simulink model "ALL_JP360_DBW_V6_5_1103"  (R2022a)
settings: Solver=FixedStepAuto  StartTime=0.0  StopTime=inf  FixedStep=0.01  RelTol=1e-3  EnableMultiTasking=on
model workspace (MAT data in the model file):
  g = 9.8
undefined symbols (not defined in the file or in its folder): canChannel, delta_v_p, IPM_Line_C0, IPM_Line_C1, IPM_Line_C2, IPM_Line_C3, M, M_p, MRR_ObjDistX, MRR_ObjDistY, MRR_ObjFusionCamID, MRR_ObjFusionSig, MRR_ObjID, MRR_ObjRelVelX, MRR_ObjRelVelY, MRR_ObjType, MRR_ObjUpdFlg, none, obj_vaild, untracktime, V, videoinput
libraries: canfdmsglib x230, canfdlib x76, slpidlib x24, simulink x18, dspstat3 x14, ctrlSharedLib x1, simulink_extras x1, imaqlib x1, realtime_pacer_lib x1, dspvision x1, visionsinks x1
(part 51 of 55)

== system ALL_JP360_DBW_V6_5_1103/ACC_Control/ACC_FUNCTION/Subsystem2/ACC_model/CC_module ==
  note: err_v＞2时根据速度段计算加速度（速度小于70mps加速度为1.5；速度大于20mps时加速度为1.3）,err_v≤2时的加速度设为0;减速度通过PID计算（速度误差0.3mps以内的减速度设为0）。
  velocity [m/s] : Inport
  Desired Velocity [m/s] : Inport  Port=2
  IC_V_kph : Inport  Port=3
  ACC_STATUSt : Inport  Port=4
  1-D Lookup Table : Lookup_n-D  NumberOfTableDimensions=1  BreakpointsForDimension1=[-2.5 -1 0 1 2 6 12 24 48 96 130]  BreakpointsForDimension2Source=Input port  Table=[-0.3 -0.1 0 0 0.8 1.5 1.7 1.8 2.0 2.0 2.2]  InternalRulePriority=Speed  RndMeth=Simplest
  1-D Lookup Table2 : Lookup_n-D  NumberOfTableDimensions=1  BreakpointsForDimension1=[-130;-96;-48;-24;-12;-6;-4;-2.5]  BreakpointsForDimension2Source=Input port  Table=[2;2;2;1;0.5;0.5;0.1;0]  InternalRulePriority=Speed  RndMeth=Simplest
  Abs2 : Abs  Commented=on  SaturateOnIntegerOverflow=off
  Add : Sum  Commented=on  Inputs=+-
  Add1 : Sum  Inputs=+-
  CalAcce : MATLAB Function  Commented=on  TreatAsAtomicUnit=on
  CalDec : slpidlib/PID Controller  Controller=PID  Form=Parallel  TimeDomain=Discrete-time  UseExternalTs=off  SampleTime=-1  IntegratorMethod=Forward Euler  FilterMethod=Forward Euler  ControllerParametersSource=external  P=1  I=1  UseKiTs=off  D=0  N=100  UseFilter=on  TunerSelectOption=Transfer Function Based (PID Tuner App)  InitialConditionSource=internal  InitialConditionForIntegrator=0  InitialConditionForFilter=0  DifferentiatorICPrevScaledInput=0  ExternalReset=either  TrackingMode=off  Kt=1  LimitOutput=off  SatLimitsSource=internal  UpperSaturationLimit=inf  LowerSaturationLimit=-inf  LinearizeAsGain=on  AntiWindupMode=none  Kb=1  POutMin=[]  POutMax=[]  IOutMin=[]  IOutMax=[]  DOutMin=[]  DOutMax=[]  NOutMin=[]  NOutMax=[]  SumOutDataTypeStr=single  SumOutMin=[]  SumOutMax=[]  SaturationOutMin=[]  SaturationOutMax=[]  PParamMin=[]  PParamMax=[]  IParamMin=[]  IParamMax=[]  DParamMin=[]  DParamMax=[]  NParamMin=[]  NParamMax=[]  KbParamMin=[]  KbParamMax=[]  KtParamMin=[]  KtParamMax=[]  KbOutMin=[]  KbOutMax=[]  KtOutMin=[]  KtOutMax=[]  IntegratorOutMin=[]  IntegratorOutMax=[]  FilterOutMin=[]  FilterOutMax=[]  SumI1OutMin=[]  SumI1OutMax=[]  SumI2OutMin=[]  SumI2OutMax=[]  SumI3OutMin=[]  SumI3OutMax=[]  SumI4OutMin=[]  SumI4OutMax=[]  SumDOutMin=[]  SumDOutMax=[]  DifferentiatorOutMin=[]  DifferentiatorOutMax=[]  FilterDiffOutCoefMin=[]  FilterDiffOutCoefMax=[]  ReciprocalOutMin=[]  ReciprocalOutMax=[]  SumDenOutMin=[]  SumDenOutMax=[]  SumNumOutMin=[]  SumNumOutMax=[]  DivideOutMin=[]  DivideOutMax=[]  UdiffTsProdOutMin=[]  UdiffTsProdOutMax=[]  NTsProdOutMin=[]  NTsProdOutMax=[]  UintegralTsProdOutMin=[]  UintegralTsProdOutMax=[]  UngainTsProdOutMin=[]  UngainTsProdOutMax=[]  IntegratorContinuousStateAttributes=''  IntegratorStateMustResolveToSignalObject=off  IntegratorRTWStateStorageClass=Auto  FilterContinuousStateAttributes=''  FilterStateMustResolveToSignalObject=off  FilterRTWStateStorageClass=Auto  ParallelPVariant=ExternalParameters  IdealPVariant=Disabled  IVariant=ExternalParameters  DVariant=ExternalParameters  IntegratorVariant=Discrete  SatVariant=Disabled  AWVariant=Passthrough  PCopyVariant=Disabled  TRVariant=Disabled  FdbkBlocksVariant=Forward  IdealPFdbkVariant=Disabled  SatFdbkVariant=Disabled  DerivativeFilterVariant=ForwardEulerFilter  NVariant=ExternalParameters  NCopyVariant=Disabled  FilterICVariant=InternalICsFilter  IntegratorICVariant=InternalICs  ExternalResetVariant=ExternalReset  TRSumVariant=Passthrough  SumFdbkVariant=Disabled  SumVariant=Sum_PID  TsampFilterVariant=InternalTs  TsampNgainVariant=Passthrough  TsampIntegralVariant=Passthrough  ExternalSaturationOutDataTypeStr=Inherit: Same as second input  aMode=0
  Constant1 : Constant  Commented=on  Value=0.01  OutDataTypeStr=single
  Constant10 : Constant  Value=100  OutDataTypeStr=int8
  Constant11 : Constant  OutDataTypeStr=single
  Constant12 : Constant  OutDataTypeStr=single
  Constant2 : Constant  Commented=on  Value=0  OutDataTypeStr=single
  Constant3 : Constant  Commented=on  Value=0  OutDataTypeStr=single
  Constant4 : Constant  Commented=on  Value=3  OutDataTypeStr=int8
  Constant{5..7,9} (4 alike) : Constant  Value=0  OutDataTypeStr=single
  Constant8 : Constant  Value=3  OutDataTypeStr=int8
  Data Type Conversion1 : DataTypeConversion  OutDataTypeStr=double  SaturateOnIntegerOverflow=off  RndMeth=Floor
  Display : Display
  From6 : From  Commented=on  GotoTag=IC_V
  Gain : Gain  Gain=3.6
  Gain1 : Gain  Gain=3.6
  Gain2 : Gain  Gain=3.6
  Gain3 : Gain  Gain=0.65
  MATLAB Function : MATLAB Function  TreatAsAtomicUnit=on
  Product : Product
  Saturation : Saturate  Commented=through  UpperLimit=1000000  LowerLimit=-10
  Saturation1 : Saturate  UpperLimit=0  LowerLimit=-2  OutDataTypeStr=single
  Saturation3 : Saturate  UpperLimit=130  LowerLimit=-2.5
  Saturation4 : Saturate  Commented=on  UpperLimit=Uplimit_acc  LowerLimit=0  OutDataTypeStr=single
  Saturation5 : Saturate  Commented=on  UpperLimit=0  LowerLimit=Uplimit_dec  OutDataTypeStr=single
  Scope : Scope  NumInputPorts=3
  Scope1 : Scope  Commented=on  NumInputPorts=3
  Sum4 : Sum  Inputs=|+-
  Switch : Switch  Threshold=-4  OutDataTypeStr=single  SaturateOnIntegerOverflow=off  InputSameDT=off
  Switch1 : Switch  Commented=on  Criteria=u2 ~= 0  SaturateOnIntegerOverflow=off  InputSameDT=off
  Switch2 : Switch  Commented=on  Criteria=u2 > Threshold  Threshold=-2.5  SaturateOnIntegerOverflow=off  InputSameDT=off
  Switch3 : Switch  Criteria=u2 ~= 0  Threshold=-0.6  SaturateOnIntegerOverflow=off  InputSameDT=off
  Switch4 : Switch  Commented=on  Criteria=u2 > Threshold  Threshold=0.3  SaturateOnIntegerOverflow=off  InputSameDT=off
  Switch5 : Switch  Threshold=-4  OutDataTypeStr=single  SaturateOnIntegerOverflow=off  InputSameDT=off
  cc_acceleration [a] : Outport
  cc_deceleration [-a] : Outport  Port=2
  wires:
  From6/1 -> CalAcce/2(IC_V)  "throttle"
  Data Type Conversion1/1 -> CalDec/1  "err_v"
  Sum4/1 -> Gain1/1, Gain/1, CalAcce/1(delta_v), Gain2/1, Saturation1/1  "err_v"
  Constant9/1 -> CalDec/4
  Constant10/1 -> CalDec/5
  velocity [m/s]/1 -> Sum4/2
  IC_V_kph/1 -> [IC_V]
  Desired Velocity [m/s]/1 -> Sum4/1
  Saturation1/1 -> Data Type Conversion1/1
  Constant2/1 -> Switch1/1
  ACC_STATUSt/1 -> [accs], Add/1
  Constant4/1 -> Add/2
  Add/1 -> Switch1/2
  Constant1/1 -> Switch1/3
  [accs] -> Add1/1
  Constant8/1 -> Add1/2
  Constant6/1 -> Switch3/1
  Product/1 -> Switch3/3  "dec"
  Add1/1 -> Switch3/2
  Switch3/1 -> MATLAB Function/3(dec_in), Display/1
  1-D Lookup Table/1 -> MATLAB Function/1(acc_in)
  ? -> Switch4/1
  Abs2/1 -> Switch4/2
  Constant3/1 -> Switch4/3
  Gain2/1 -> Switch5/2, Switch/2, 1-D Lookup Table2/1
  1-D Lookup Table2/1 -> Gain3/1
  ? -> Scope1/3
  Saturation4/1 -> Scope1/1
  Saturation5/1 -> Scope1/2
  Switch2/1 -> Saturation4/1, Saturation5/1
  Gain1/1 -> Scope/2, MATLAB Function/2(delta_v)
  MATLAB Function/1(acc_out) -> Saturation/1
  MATLAB Function/2(dec_out) -> cc_deceleration [-a]/1, Scope/3
  Gain/1 -> Saturation3/1
  Saturation3/1 -> 1-D Lookup Table/1
  Switch/1 -> CalDec/3
  Constant5/1 -> Switch/1
  Constant7/1 -> Switch/3
  Saturation/1 -> cc_acceleration [a]/1, Scope/1
  Constant12/1 -> Switch5/1
  Constant11/1 -> Switch5/3
  Switch5/1 -> Product/2
  CalDec/1 -> Product/1  "dec"
  Gain3/1 -> CalDec/2

== system ALL_JP360_DBW_V6_5_1103/ACC_Control/ACC_FUNCTION/Subsystem2/ACC_model/Rate transition from other signals1 ==
  In1 : Inport
  In2 : Inport  Port=2
  Rate Transition1 : RateTransition  Integrity=off  OutPortSampleTime=Tsensor
  Rate Transition2 : RateTransition  Integrity=off  OutPortSampleTime=Tsensor
  Out1 : Outport
  Out2 : Outport  Port=2
  wires:
  Rate Transition2/1 -> Out2/1
  In2/1 -> Rate Transition2/1
  Rate Transition1/1 -> Out1/1
  In1/1 -> Rate Transition1/1

== system ALL_JP360_DBW_V6_5_1103/ACC_Control/ACC_FUNCTION/Subsystem2/ACC_model/Rate transition from EGO1 ==
  In1 : Inport
  In2 : Inport  Port=2
  Des_speed[m/s]1 : Inport  Port=3
  abs_speed[m/s]1 : Inport  Port=4
  abs_speed[m/s]2 : Inport  Port=5
  Des_speed[m/s]2 : Inport  Port=6
  Des_speed[m/s]3 : Inport  Port=7
  Rate Transition{1..7} (7 alike) : RateTransition  Integrity=off  OutPortSampleTime=Tsensor
  Out1 : Outport
  Out2 : Outport  Port=2
  Out3 : Outport  Port=3
  Out4 : Outport  Port=4
  Out5 : Outport  Port=5
  Out6 : Outport  Port=6
  Out7 : Outport  Port=7
  wires:
  In1/1 -> Rate Transition1/1
  Rate Transition1/1 -> Out1/1
  In2/1 -> Rate Transition2/1
  Rate Transition2/1 -> Out2/1
  Rate Transition3/1 -> Out3/1
  Des_speed[m/s]1/1 -> Rate Transition3/1
  Rate Transition5/1 -> Out5/1
  Rate Transition4/1 -> Out4/1
  abs_speed[m/s]2/1 -> Rate Transition5/1
  abs_speed[m/s]1/1 -> Rate Transition4/1
  Des_speed[m/s]2/1 -> Rate Transition6/1
  Rate Transition6/1 -> Out6/1
  Rate Transition7/1 -> Out7/1
  Des_speed[m/s]3/1 -> Rate Transition7/1

== system ALL_JP360_DBW_V6_5_1103/ACC_Control/ACC_FUNCTION/Subsystem2/ACC_model/Rate transition from TIS2 ==
  In1 : Inport
  In2 : Inport  Port=2
  Rate Transition1 : RateTransition  Integrity=off  OutPortSampleTime=Tsensor
  Rate Transition2 : RateTransition  Integrity=off  OutPortSampleTime=Tsensor
  Out1 : Outport
  Out2 : Outport  Port=2
  wires:
  Rate Transition2/1 -> Out2/1
  In2/1 -> Rate Transition2/1
  Rate Transition1/1 -> Out1/1
  In1/1 -> Rate Transition1/1

== system ALL_JP360_DBW_V6_5_1103/ACC_Control/ACC_FUNCTION/Subsystem2/ACC_model/TIS1 ACC action ==
  note: === 避撞模式说明 ===
      |
      |  - ACC_MODE: 0, 未知模式
      |  - ACC_MODE: 1, 表示避撞模式
      |  - ACC_MODE: 2, 定速巡航模式
      |  - ACC_MODE: 3, 跟进模式
      |  - ACC_MODE: 4, 跟车模式
  note: === TIS1 ACC action block ===
      |
      |  - control block,
      |  - uses information provided by the first sensor,
      |  - limits acceleration and deceleration of the EGO car,
      |  - adjusts throttle and brake pressure of the EGO car,
      |  - the control strategy is to maintain HeadWay Time (HWT)
      |    on desirable level.
  v_ego : Inport
  v_obj : Inport  Port=2
  d_obj : Inport  Port=3
  cc_acceleration_in : Inport  Port=4
  cc_deceleration_in : Inport  Port=5
  v_set : Inport  Port=6
  t_dem : Inport  Port=7
  standstill : Inport  Port=8
  obj_detacted_flag : Inport  Port=9
  Subsystem1 : Subsystem
  acceleration[a] : Outport
  deceleration[-a] : Outport  Port=2
  ACC_MODE : Outport  Port=3
  standstill_req : Outport  Port=4  InitialOutput=[150]
  wires:
  cc_acceleration_in/1 -> Subsystem1/7(cc_throttle)
  obj_detacted_flag/1 -> Subsystem1/9(obj_detcted_flag)
  cc_deceleration_in/1 -> Subsystem1/8(cc_brake)
  standstill/1 -> Subsystem1/6(standstill)
  t_dem/1 -> Subsystem1/5(t_dem)
  v_set/1 -> Subsystem1/4(v_set)
  d_obj/1 -> Subsystem1/3(d_obj)
  v_obj/1 -> Subsystem1/2(v_obj)
  v_ego/1 -> Subsystem1/1(v_ego)
  Subsystem1/1(acceleration [a]) -> acceleration[a]/1
  Subsystem1/2(deceleration [-a]) -> deceleration[-a]/1
  Subsystem1/3(ACC_MODE) -> ACC_MODE/1
  Subsystem1/4(standstill_req) -> standstill_req/1

== system ALL_JP360_DBW_V6_5_1103/ACC_Control/ACC_FUNCTION/Subsystem2/ACC_model/calculate_slope ==
  note: Pitch_angle为正值时表示抬头
      | Pitch_angle为负值时表示低头
      | 抬头表示上坡
      | 低头表示下坡
      |
      | MP5 0*544有pitch真值
  ax_esp : Inport
  ω : Inport  Port=2
  δ : Inport  Port=3
  vx1 : Inport  Port=4
  Add{,1..4} (5 alike) : Sum  Commented=on  Inputs=+-
  Add5 : Sum  Inputs=+-
  Add6 : Sum  Inputs=+-
  Asin : Trigonometry  Commented=on  Operator=asin
  Asin1 : Trigonometry  Operator=asin
  Constant : Constant  Value=9.8  VectorParams1D=off  OutDataTypeStr=single  SampleTime=-1
  Cos : Trigonometry  Commented=on  Operator=cos
  Delay : Delay  Commented=on  DelayLength=1  InitialCondition=0  UseCircularBuffer=on
  Delay1 : Delay  Commented=on  DelayLength=1  InitialCondition=0  UseCircularBuffer=on
  Delay2 : Delay  DelayLength=1  InitialCondition=0  UseCircularBuffer=on
  Divide : Product  Commented=on  Inputs=*/
  Divide1 : Product  Commented=on  Inputs=**/**
  Divide2 : Product  Commented=on  Inputs=***
  Divide3 : Product  Commented=on  Inputs=*/
  Divide4 : Product  Commented=on  Inputs=*/
  Divide5 : Product  Commented=on  Inputs=**
  Divide6 : Product  Commented=on  Inputs=/*
  Divide7 : Product  Inputs=*/
  Gain1 : Gain  Commented=on  Gain=57.3
  Gain2 : Gain  Gain=57.3
  L : Constant  Commented=on  OutDataTypeStr=single
  Median Filter1 : dspstat3/Median Filter  WindowLength=20  SimulateUsing=Interpreted execution
      settings: SourceProductBaseCode=DS
  Median Filter2 : dspstat3/Median Filter  WindowLength=20  SimulateUsing=Interpreted execution
      settings: SourceProductBaseCode=DS
  Moving Average : dspstat3/Moving Average  Commented=on  Method=Sliding window  ForgettingFactorPort=off  SpecifyWindowLength=on  WindowLength=Moving_Average_Window  ForgettingFactor=0.9  SimulateUsing=Code generation
  Rate Transition : RateTransition
  Recursive Least Squares Estimator : ctrlSharedLib/Recursive Least Squares Estimator  InitialEstimateSource=None  InitialParameterData=1  P0=1e4  InitialRegressors=0  InitialOutputs=0  History=Infinite  WindowLength=200  EstimationMethod=Forgetting Factor  AdaptationParameter=0.95  HasTimeVaryingAdaptationParameter=off  NormalizationBias=eps  OutputError=off  OutputP=off  AddEnablePort=off  InputProcessing=Sample-based  Ts=0.01
      settings: SourceProductBaseCode=CT,ID
  Saturation : Saturate  Commented=on  UpperLimit=1  LowerLimit=-1
  Scope : Scope  Commented=on  NumInputPorts=3
  Scope1 : Scope  Commented=on  NumInputPorts=2
  Scope2 : Scope  Commented=on
  Scope3 : Scope
  Scope4 : Scope
  Scope6 : Scope
  Sin : Trigonometry  Commented=on
  Square : Math  Commented=on  Operator=square
  Switch : Switch  Commented=on  Criteria=u2 > Threshold  SaturateOnIntegerOverflow=off  InputSameDT=off
  Switch1 : Switch  Commented=on  Criteria=u2 > Threshold  SaturateOnIntegerOverflow=off  InputSameDT=off
  Z : Constant  Commented=on  OutDataTypeStr=single
  g : Constant  Commented=on  Value=9.81  OutDataTypeStr=single
  g1 : Constant  Commented=on  Value=9.81  OutDataTypeStr=single
  Φ : Constant  Commented=on  OutDataTypeStr=single
  仿真步长 : Constant  Commented=on  Value=0.01  OutDataTypeStr=single
  仿真步长1 : Constant  Value=0.01  OutDataTypeStr=single
  φ : Outport
  wires:
  vx1/1 -> Delay2/1, Add6/1
  Delay2/1 -> Add6/2
  仿真步长1/1 -> Divide7/2
  Add6/1 -> Divide7/1
  Gain2/1 -> Scope3/1
  Constant/1 -> Recursive Least Squares Estimator/1
  Recursive Least Squares Estimator/1 -> Asin1/1
  Add5/1 -> Rate Transition/1, Scope6/1
  [ax_esp] -> Median Filter2/1
  Asin1/1 -> Gain2/1, φ/1
  Median Filter2/1 -> Scope4/1, Add5/1
  Divide7/1 -> Median Filter1/1
  Median Filter1/1 -> Add5/2
  Gain1/1 -> Scope2/1
  Switch1/1 -> Scope/3
  Moving Average/1 -> Add/1, Add1/1, Scope1/1
  Add4/1 -> Divide3/1
  仿真步长/1 -> Divide3/2
  Divide3/1 -> Divide1/5, Add/2, Scope/2, Scope1/2
  Delay1/1 -> Add4/2
  g1/1 -> Divide4/2, Divide5/2
  Add3/1 -> Divide/1
  Square/1 -> Divide1/2, Divide2/3
  ax_esp/1 -> Moving Average/1, Scope/1
  Φ/1 -> Sin/1, Cos/1
  Cos/1 -> Divide2/2
  Sin/1 -> Divide1/1
  Asin/1 -> Switch/1  "转向"
  Add1/1 -> Add3/1
  Divide2/1 -> Add3/2
  Z/1 -> Divide1/4
  ω/1 -> Square/1
  L/1 -> Divide2/1
  δ/1 -> Switch/2
  Divide4/1 -> Divide5/1  "β"
  Divide6/1 -> Saturation/1
  Delay/1 -> Switch1/3
  Saturation/1 -> Add2/1
  Divide/1 -> Asin/1
  ? -> Add4/1, Delay1/1, Switch1/2, Divide1/3
  Add2/1 -> Delay/1, Switch1/1  "行车"
  Add/1 -> Divide4/1, Divide6/2
  Divide5/1 -> Switch/3  "直行"
  Switch/1 -> Add2/2  "β"
  Divide1/1 -> Add1/2
  g/1 -> Divide6/1, Divide/2
  Rate Transition/1 -> Recursive Least Squares Estimator/2

== system ALL_JP360_DBW_V6_5_1103/ACC_Control/ACC_FUNCTION/Subsystem2/ACC_model/curve agl ==
  yaw_rate : Inport
  ay_esp : Inport  Port=2
  desire_speed : Inport  Port=3
  Abs1 : Abs  SaturateOnIntegerOverflow=off
  Abs2 : Abs  SaturateOnIntegerOverflow=off
  Add2 : Sum  Inputs=-+
  Add3 : Sum  Inputs=-+
  Divide : Product  Inputs=*/  RndMeth=Zero  SaturateOnIntegerOverflow=on
  Gain4 : Gain  Gain=1/57.3
  Moving Average : dspstat3/Moving Average  Method=Sliding window  ForgettingFactorPort=off  SpecifyWindowLength=on  WindowLength=Moving_Average_Window  ForgettingFactor=0.9  SimulateUsing=Code generation
  Relational Operator : RelationalOperator  Operator=<=  OutDataTypeStr=boolean  RndMeth=Simplest  InputSameDT=off
  Saturation2 : Saturate  UpperLimit=3  LowerLimit=0.05
  Switch1 : Switch  Criteria=u2 > Threshold  Threshold=0.5  OutDataTypeStr=single  SaturateOnIntegerOverflow=off  InputSameDT=off
  Switch2 : Switch  Criteria=u2 > Threshold  SaturateOnIntegerOverflow=off  InputSameDT=off
  curv_k : Gain
  Output : Outport
  wires:
  Moving Average/1 -> Abs2/1
  ay_esp/1 -> Moving Average/1
  yaw_rate/1 -> Abs1/1
  Gain4/1 -> Divide/2
  Switch2/1 -> Add2/1
  Add2/1 -> curv_k/1
  Abs1/1 -> Saturation2/1, Switch1/2
  Add3/1 -> Switch1/1
  curv_k/1 -> Add3/1
  Switch1/1 -> Output/1
  desire_speed/1 -> Relational Operator/2, Switch2/3, Switch1/3, Add3/2, Add2/2
  Relational Operator/1 -> Switch2/2
  Abs2/1 -> Divide/1
  Divide/1 -> Relational Operator/1, Switch2/1
  Saturation2/1 -> Gain4/1

== system ALL_JP360_DBW_V6_5_1103/ACC_Control/ACC_FUNCTION/Subsystem2/Limit/a2m_表达式 ==
  slope : Inport
  acce : Inport  Port=2
  dec : Inport  Port=3
  velocity_abs : Inport  Port=4
  Add : Sum  Inputs=++++
  Add1 : Sum
  Constant3 : Constant  Value=mass
  Gain : Gain  Gain=Width*Hight
  Gain1 : Gain  Gain=1/21.15
  Gain2 : Gain  Gain=mass
  Gain3 : Gain  Gain=thgma_total
  Gain4 : Gain  Gain=r_tire
  Gain5 : Gain  Gain=C_fk
  Gain6 : Gain  Gain=g
  Gain7 : Gain  Gain=0.1
  Gain8 : Gain  Gain=0.08
  Math Function : Math  Operator=square
  Product : Product
  Product1 : Product
  Product2 : Product
  Saturation1 : Saturate  UpperLimit=0  LowerLimit=-6
  滚动阻力系数 : Constant  Value=C_f0
  风阻系数 : Constant  Value=C_d
  throttle[NM] : Outport
  brake[-a] : Outport  Port=2
  wires:
  Gain8/1 -> Add/1
  Gain7/1 -> Add/4
  slope/1 -> Product1/1
  Gain4/1 -> throttle[NM]/1
  dec/1 -> Saturation1/1
  Saturation1/1 -> brake[-a]/1
  Add/1 -> Gain4/1
  Gain3/1 -> Gain8/1
  Gain2/1 -> Gain3/1
  acce/1 -> Gain2/1
  Product2/1 -> Add/2
  Math Function/1 -> Product2/1
  Gain1/1 -> Product2/2
  Gain/1 -> Gain1/1
  风阻系数/1 -> Gain/1
  Product1/1 -> Add/3
  Product/1 -> Gain7/1
  Constant3/1 -> Gain6/1
  Gain6/1 -> Product/1, Product1/2
  滚动阻力系数/1 -> Add1/2
  Gain5/1 -> Add1/1
  Add1/1 -> Product/2
  velocity_abs/1 -> Gain5/1, Math Function/1

== system ALL_JP360_DBW_V6_5_1103/ACC_Control/ACC_FUNCTION/Subsystem2/Limit/a2m_表达式_标定表 ==
  acce : Inport
  IC_V_kph : Inport  Port=2
  slope : Inport  Port=3
  ACC_STATUSt : Inport  Port=4
  Set_speed_mps1 : Inport  Port=5
  abs_mps1 : Inport  Port=6
  dec_m : Inport  Port=7
  1-D Lookup Table : Lookup_n-D  NumberOfTableDimensions=1  BreakpointsForDimension1=V  BreakpointsForDimension2Source=Input port  Table=M  InternalRulePriority=Speed  RndMeth=Simplest
  Add : Sum  Inputs=+-
  Add1 : Sum  Inputs=++++  AccumDataTypeStr=single  OutDataTypeStr=single
  Add4 : Sum  Inputs=+-
  Constant1 : Constant  OutDataTypeStr=single
  Constant3 : Constant  Commented=on  Value=10  OutDataTypeStr=single
  Constant4 : Constant  Value=3  OutDataTypeStr=int8
  Constant5 : Constant  Value=0  OutDataTypeStr=single
  Constant6 : Constant  Commented=on  Value=100  OutDataTypeStr=single
  Data Type Conversion1 : DataTypeConversion  OutDataTypeStr=single  SaturateOnIntegerOverflow=off  RndMeth=Floor
  From1 : From  Commented=on  GotoTag=delta_v
  From2 : From  Commented=on  GotoTag=delta_v
  From3 : From  Commented=on  GotoTag=delta_v
  Gain1 : Gain  Gain=g
  Gain10 : Gain  Gain=0
  Gain2 : Gain  Gain=mass
  Gain3 : Gain  Gain=thgma_total
  Gain4 : Gain  Gain=r_tire
  Gain5 : Gain  Gain=mass
  Gain6 : Gain  Gain=r_tire
  Gain7 : Gain  Gain=0.06
  Gain8 : Gain  Gain=0.06
  MATLAB Function : MATLAB Function  Commented=on  TreatAsAtomicUnit=on
  Manual Switch : ManualSwitch
  Rate Limiter : RateLimiter  RisingSlewLimit=50  FallingSlewLimit=-50  SampleTimeMode=inherited
  Rate Limiter2 : RateLimiter  Commented=through  RisingSlewLimit=60  FallingSlewLimit=-20  SampleTimeMode=inherited
  Relay : Relay  Commented=on
  Scope : Scope
  Scope1 : Scope  NumInputPorts=2
  Subsystem : Subsystem  Commented=on
  Subsystem1 : Subsystem  Commented=on
  Switch : Switch  Criteria=u2 ~= 0  SaturateOnIntegerOverflow=off  InputSameDT=off
  Switch1 : Switch  Commented=on  Criteria=u2 > Threshold  Threshold=-2.5  SaturateOnIntegerOverflow=off  InputSameDT=off
  T_PID : Subsystem
  throttle[NM] : Outport
  M_slope : Outport  Port=2
  M_a : Outport  Port=3
  M_cc : Outport  Port=4
  M_pid : Outport  Port=5
  wires:
  Gain7/1 -> Add1/2, M_a/1
  Gain8/1 -> Gain10/1
  Gain3/1 -> Gain2/1
  Rate Limiter/1 -> Gain5/1
  Gain6/1 -> Gain8/1
  Gain5/1 -> Gain6/1
  Gain4/1 -> Gain7/1
  1-D Lookup Table/1 -> Add1/3, M_cc/1
  Gain2/1 -> Gain4/1
  Gain1/1 -> Rate Limiter/1
  slope/1 -> Gain1/1
  IC_V_kph/1 -> Data Type Conversion1/1  "throttle"
  Data Type Conversion1/1 -> 1-D Lookup Table/1
  Add1/1 -> throttle[NM]/1, Scope/1
  acce/1 -> Gain3/1
  Constant4/1 -> Add/2
  ACC_STATUSt/1 -> [accs], Add/1
  Add/1 -> Switch/2
  Constant5/1 -> Switch/1
  Constant1/1 -> Switch/3
  Constant6/1 -> MATLAB Function/3(p2)
  Constant3/1 -> MATLAB Function/2(p1)
  Gain10/1 -> Add1/1, M_slope/1
  abs_mps1/1 -> Add4/2
  Set_speed_mps1/1 -> Add4/1
  Add4/1 -> [delta_v]
  Rate Limiter2/1 -> M_pid/1, Add1/4, Scope1/1
  Switch/1 -> [PIDstatus]
  From2/1 -> Subsystem/1(In2)
  From1/1 -> Subsystem1/1(In1)
  From3/1 -> Switch1/2
  Manual Switch/1 -> Scope1/2, Rate Limiter2/1
  Subsystem/1(throttle) -> Switch1/1
  Subsystem1/1(Out1) -> Switch1/3
  Switch1/1 -> Manual Switch/2
  T_PID/1(throttle) -> Manual Switch/1
  [delta_v] -> T_PID/1(In1)
  [accs] -> T_PID/2(ACC_STATUSt1)
  dec_m/1 -> [dec_m]
  [dec_m] -> T_PID/3(dec_m)

== system ALL_JP360_DBW_V6_5_1103/ACC_Control/ACC_FUNCTION/Subsystem2/Limit/acceleration_throttle——PID ==
  note: 设定车速，3pid分段
  dec : Inport
  setvalue : Inport  Port=2
  acce1 : Inport  Port=3
  IC_V_kph : Inport  Port=4
  If : If
  Manual Switch : ManualSwitch
  Merge2 : Merge
  Out_PID : Subsystem
  Saturation1 : Saturate  UpperLimit=0  LowerLimit=-8
  Subsystem1 : Subsystem
  Subsystem2 : Subsystem
  brake[-a] : Outport
  throttle[a]1 : Outport  Port=2
  wires:
  Manual Switch/1 -> throttle[a]1/1
  Merge2/1 -> Manual Switch/2
  acce1/1 -> Out_PID/1(acce), [a]
  [setv] -> Subsystem2/2(setv)
  [setv] -> If/1
  [a] -> Subsystem2/1(acce)
  setvalue/1 -> Out_PID/3(setvalue), [setv]
  Subsystem2/1(Out1) -> Merge2/1
  Subsystem1/1(Out1) -> Merge2/2
  If/1 -> Subsystem2/Action
  If/2 -> Subsystem1/Action
  Out_PID/1(throttle[a]1) -> Manual Switch/1
  IC_V_kph/1 -> Out_PID/2(IC_V_kph)
  dec/1 -> Saturation1/1
  Saturation1/1 -> brake[-a]/1

== system ALL_JP360_DBW_V6_5_1103/ACC_Control/ACC_FUNCTION/Subsystem2/ACC_model/TIS1 ACC action/Subsystem1 ==
  v_ego : Inport
  v_obj : Inport  Port=2
  d_obj : Inport  Port=3
  v_set : Inport  Port=4
  t_dem : Inport  Port=5
  standstill : Inport  Port=6
  cc_throttle : Inport  Port=7
  cc_brake : Inport  Port=8
  obj_detcted_flag : Inport  Port=9
  Add : Sum
  Add1 : Sum
  Constant : Constant  Value=0
  Data Type Conversion : DataTypeConversion  OutDataTypeStr=int8  SaturateOnIntegerOverflow=off  RndMeth=Floor
  Data Type Conversion1 : DataTypeConversion  OutDataTypeStr=single  SaturateOnIntegerOverflow=off  RndMeth=Floor
  Demux : Demux  Outputs=3
  Display : Display
  Divide : Product  Inputs=*/
  Math Function : Math  Operator=square
  Math Function1 : Math  Operator=square
  Merge : Merge
  Mux : Mux  Inputs=3
  Mux2 : Mux  Inputs=3
  Product1 : Product
  Product8 : Product
  Scope : Scope  NumInputPorts=4
  Scope1 : Scope  NumInputPorts=3
  Subtract{,1..4,8..9} (7 alike) : Sum  Inputs=+-
  Subtract5 : Sum
  Switch : Switch  Criteria=u2 > Threshold  SaturateOnIntegerOverflow=off  InputSameDT=off
  To Workspace : ToWorkspace  VariableName=azero  SaveFormat=Timeseries  SampleTime=-1
  To Workspace1 : ToWorkspace  VariableName=delta_d_ego  SaveFormat=Timeseries  SampleTime=-1
  a_max1 : Constant  Value=-6  OutDataTypeStr=single
  collision : Subsystem  TreatAsAtomicUnit=on
  if : If
  k3 : Gain  Gain=0.2
  k4 : Gain  Gain=0.8
  mode change : Subsystem  TreatAsAtomicUnit=on
  t_yanshi : Gain  Gain=0.4
  acceleration [a] : Outport
  deceleration [-a] : Outport  Port=2
  ACC_MODE : Outport  Port=3
  standstill_req : Outport  Port=4  InitialOutput=[150]
  wires:
  [delta_d_ego] -> Data Type Conversion1/1
  Subtract5/1 -> [v_obj]
  [v_ego] -> Subtract5/2
  Subtract8/1 -> Subtract9/1
  t_yanshi/1 -> Add/2
  Subtract/1 -> t_yanshi/1
  [t_dem] -> Scope/3, Product1/1
  a_max1/1 -> Divide/2
  [d] -> Subtract3/1, Scope/1
  [t_dem] -> Product8/1
  [v_obj] -> Product8/2
  [d0] -> Subtract4/2
  Subtract9/1 -> [delta_d_obj]
  [d0] -> Subtract9/2
  Product8/1 -> Subtract8/2
  [d] -> Subtract8/1
  Math Function1/1 -> Subtract1/2
  [v_obj] -> Math Function1/1
  Math Function/1 -> Subtract1/1
  Product1/1 -> Subtract3/2, Scope/2
  [v_obj_relative] -> Scope1/3, [delta_v], Subtract5/1  "delta_v"
  [v_ego] -> Product1/2, Scope/4
  Divide/1 -> Add/1
  Subtract4/1 -> Scope1/1, To Workspace1/1, [delta_d_ego]  "delta_d_ego"
  [v_ego] -> Math Function/1
  Add/1 -> Subtract2/1
  [d] -> Subtract2/2
  [v_obj] -> Subtract/2
  Subtract3/1 -> Subtract4/1
  [v_ego] -> Subtract/1
  Subtract1/1 -> Divide/1
  v_ego/1 -> [v_ego]
  v_obj/1 -> [v_obj_relative]
  v_set/1 -> [v_set]
  d_obj/1 -> [d]
  t_dem/1 -> [t_dem]
  standstill/1 -> [d0]
  Demux/2 -> deceleration [-a]/1
  Mux2/1 -> Merge/2
  Mux/1 -> Merge/1
  if/2 -> mode change/Action
  collision/2(deceleration [-a]) -> Mux/2
  if/1 -> collision/Action
  collision/1(acceleration [a]) -> Mux/1
  Merge/1 -> Demux/1
  Demux/1 -> acceleration [a]/1
  mode change/1(acceleration [a]) -> Mux2/1
  mode change/2(deceleration [-a]) -> Mux2/2
  cc_throttle/1 -> mode change/1(cc_throttle)
  cc_brake/1 -> mode change/2(cc_brake)
  obj_detcted_flag/1 -> mode change/3(acc_obj_detected), Switch/2
  k3/1 -> Add1/1
  k4/1 -> Add1/2
  [delta_v] -> k4/1
  Add1/1 -> [a_zero], Scope1/2, To Workspace/1  "a_zero"
  [a_zero] -> mode change/4(a_zero)
  [v_obj] -> mode change/5(v_obj)
  [delta_d_ego] -> mode change/8(delta_d_ego)
  mode change/3(ACC_MODE) -> Mux2/3
  collision/3(ACC_MODE) -> Mux/3
  Demux/3 -> Data Type Conversion/1
  Subtract2/1 -> Switch/1
  Switch/1 -> if/1
  Constant/1 -> Switch/3
  mode change/4(standstill_req) -> standstill_req/1
  [v_set] -> mode change/6(v_set)
  [v_ego] -> mode change/7(v_ego)
  Data Type Conversion/1 -> ACC_MODE/1, Display/1
  Data Type Conversion1/1 -> k3/1
  [d] -> mode change/9(dx)

== system ALL_JP360_DBW_V6_5_1103/ACC_Control/ACC_FUNCTION/Subsystem2/Limit/a2m_表达式_标定表/Subsystem ==
  In2 : Inport
  Abs : Abs  SaturateOnIntegerOverflow=off
  Constant : Constant  Value=100  OutDataTypeStr=int8
  Constant1 : Constant  Value=0  OutDataTypeStr=single
  Constant2 : Constant  Value=0  OutDataTypeStr=single
  Constant7 : Constant  Value=2.5  OutDataTypeStr=single
  Constant8 : Constant  Value=200  OutDataTypeStr=uint8
  Constant9 : Constant  OutDataTypeStr=single
  Gain : Gain  Gain=3.6
  PID Controller1 : slpidlib/PID Controller  Controller=PID  Form=Parallel  TimeDomain=Discrete-time  UseExternalTs=off  SampleTime=-1  IntegratorMethod=Forward Euler  FilterMethod=Forward Euler  ControllerParametersSource=external  P=1  I=1  UseKiTs=off  D=0  N=100  UseFilter=on  TunerSelectOption=Transfer Function Based (PID Tuner App)  InitialConditionSource=internal  InitialConditionForIntegrator=0  InitialConditionForFilter=0  DifferentiatorICPrevScaledInput=0  ExternalReset=none  TrackingMode=off  Kt=1  LimitOutput=off  SatLimitsSource=internal  UpperSaturationLimit=inf  LowerSaturationLimit=-inf  LinearizeAsGain=on  AntiWindupMode=none  Kb=1  PGainOutDataTypeStr=single  PProdOutDataTypeStr=single  POutMin=[]  POutMax=[]  IGainOutDataTypeStr=single  IProdOutDataTypeStr=single  IOutMin=[]  IOutMax=[]  DGainOutDataTypeStr=single  DProdOutDataTypeStr=single  DOutMin=[]  DOutMax=[]  NGainOutDataTypeStr=single  NProdOutDataTypeStr=single  NOutMin=[]  NOutMax=[]  SumOutDataTypeStr=single  SumOutMin=[]  SumOutMax=[]  SaturationOutMin=[]  SaturationOutMax=[]  PParamMin=[]  PParamMax=[]  IParamMin=[]  IParamMax=[]  DParamMin=[]  DParamMax=[]  NParamMin=[]  NParamMax=[]  KbParamMin=[]  KbParamMax=[]  KtParamMin=[]  KtParamMax=[]  KbOutMin=[]  KbOutMax=[]  KtOutMin=[]  KtOutMax=[]  IntegratorOutMin=[]  IntegratorOutMax=[]  FilterOutMin=[]  FilterOutMax=[]  SumI1OutMin=[]  SumI1OutMax=[]  SumI2OutMin=[]  SumI2OutMax=[]  SumI3OutMin=[]  SumI3OutMax=[]  SumI4OutMin=[]  SumI4OutMax=[]  SumDOutMin=[]  SumDOutMax=[]  DifferentiatorOutMin=[]  DifferentiatorOutMax=[]  FilterDiffOutCoefMin=[]  FilterDiffOutCoefMax=[]  ReciprocalOutMin=[]  ReciprocalOutMax=[]  SumDenOutMin=[]  SumDenOutMax=[]  SumNumOutMin=[]  SumNumOutMax=[]  DivideOutMin=[]  DivideOutMax=[]  UdiffTsProdOutMin=[]  UdiffTsProdOutMax=[]  NTsProdOutMin=[]  NTsProdOutMax=[]  UintegralTsProdOutMin=[]  UintegralTsProdOutMax=[]  UngainTsProdOutMin=[]  UngainTsProdOutMax=[]  IntegratorContinuousStateAttributes=''  IntegratorStateMustResolveToSignalObject=off  IntegratorRTWStateStorageClass=Auto  FilterContinuousStateAttributes=''  FilterStateMustResolveToSignalObject=off  FilterRTWStateStorageClass=Auto  ParallelPVariant=ExternalParameters  IdealPVariant=Disabled  IVariant=ExternalParameters  DVariant=ExternalParameters  IntegratorVariant=Discrete  SatVariant=Disabled  AWVariant=Passthrough  PCopyVariant=Disabled  TRVariant=Disabled  FdbkBlocksVariant=Forward  IdealPFdbkVariant=Disabled  SatFdbkVariant=Disabled  DerivativeFilterVariant=ForwardEulerFilter  NVariant=ExternalParameters  NCopyVariant=Disabled  FilterICVariant=InternalICsFilter  IntegratorICVariant=InternalICs  ExternalResetVariant=Disabled  TRSumVariant=Passthrough  SumFdbkVariant=Disabled  SumVariant=Sum_PID  TsampFilterVariant=InternalTs  TsampNgainVariant=Passthrough  TsampIntegralVariant=Passthrough  ExternalSaturationOutDataTypeStr=Inherit: Same as second input  aMode=0
  Relational Operator : RelationalOperator  Operator=<=  OutDataTypeStr=boolean  RndMeth=Simplest  InputSameDT=off
  Saturation : Saturate  UpperLimit=1  LowerLimit=-1
  Switch1 : Switch  Criteria=u2 ~= 0  SaturateOnIntegerOverflow=off  InputSameDT=off
  throttle : Outport
  wires:
  In2/1 -> Saturation/1, Abs/1
  Saturation/1 -> PID Controller1/1
  Constant8/1 -> PID Controller1/2
  Constant2/1 -> PID Controller1/4
  Abs/1 -> Gain/1
  Constant7/1 -> Relational Operator/2
  Gain/1 -> Relational Operator/1
  Constant/1 -> PID Controller1/5
  Constant9/1 -> Switch1/3
  Relational Operator/1 -> Switch1/2
  Switch1/1 -> PID Controller1/3
  PID Controller1/1 -> throttle/1  "throttle"
  Constant1/1 -> Switch1/1

== system ALL_JP360_DBW_V6_5_1103/ACC_Control/ACC_FUNCTION/Subsystem2/Limit/a2m_表达式_标定表/Subsystem1 ==
  In1 : Inport
  1-D Lookup Table1 : Lookup_n-D  NumberOfTableDimensions=1  BreakpointsForDimension1=delta_v_p  BreakpointsForDimension2Source=Input port  Table=M_p  InternalRulePriority=Speed  RndMeth=Simplest
  Out1 : Outport
  wires:
  In1/1 -> 1-D Lookup Table1/1
  1-D Lookup Table1/1 -> Out1/1

== system ALL_JP360_DBW_V6_5_1103/ACC_Control/ACC_FUNCTION/Subsystem2/Limit/a2m_表达式_标定表/T_PID ==
  In1 : Inport
  ACC_STATUSt1 : Inport  Port=2
  dec_m : Inport  Port=3
  1-D Lookup Table1 : Lookup_n-D  NumberOfTableDimensions=1  BreakpointsForDimension1=delta_v_p  BreakpointsForDimension2Source=Input port  Table=M_p  InternalRulePriority=Speed  RndMeth=Simplest
  AND : Logic  IconShape=distinctive  AllPortsSameDT=off  OutDataTypeStr=boolean
  Abs : Abs  SaturateOnIntegerOverflow=off
  Add2 : Sum  Inputs=+-
  Add3 : Sum  Inputs=+-
  Constant : Constant  Value=100  OutDataTypeStr=int8
  Constant{1,3,7,10,12..13,17} (7 alike) : Constant  Value=0  OutDataTypeStr=single
  Constant11 : Constant  Value=3  OutDataTypeStr=int8
  Constant15 : Constant  Value=2.5  OutDataTypeStr=single
  Constant16 : Constant  Value=50  OutDataTypeStr=uint8
  Constant2 : Constant  Value=8  OutDataTypeStr=single
  Constant4 : Constant  Value=-2.5  OutDataTypeStr=single
  Constant9 : Constant  Value=3  OutDataTypeStr=int8
  Display : Display
  Display1 : Display
  Gain : Gain  Gain=3.6
  Gain11 : Gain  Gain=3.6
  Gain9 : Gain  Gain=3.6
  PID Controller1 : slpidlib/PID Controller  Controller=PID  Form=Parallel  TimeDomain=Discrete-time  UseExternalTs=off  SampleTime=-1  IntegratorMethod=Forward Euler  FilterMethod=Forward Euler  ControllerParametersSource=external  P=1  I=1  UseKiTs=off  D=0  N=100  UseFilter=on  TunerSelectOption=Transfer Function Based (PID Tuner App)  InitialConditionSource=internal  InitialConditionForIntegrator=0  InitialConditionForFilter=0  DifferentiatorICPrevScaledInput=0  ExternalReset=either  TrackingMode=off  Kt=1  LimitOutput=off  SatLimitsSource=internal  UpperSaturationLimit=inf  LowerSaturationLimit=-inf  LinearizeAsGain=on  AntiWindupMode=none  Kb=1  PGainOutDataTypeStr=single  PProdOutDataTypeStr=single  POutMin=[]  POutMax=[]  IGainOutDataTypeStr=single  IProdOutDataTypeStr=single  IOutMin=[]  IOutMax=[]  DGainOutDataTypeStr=single  DProdOutDataTypeStr=single  DOutMin=[]  DOutMax=[]  NGainOutDataTypeStr=single  NProdOutDataTypeStr=single  NOutMin=[]  NOutMax=[]  SumOutDataTypeStr=single  SumOutMin=[]  SumOutMax=[]  SaturationOutMin=[]  SaturationOutMax=[]  PParamMin=[]  PParamMax=[]  IParamMin=[]  IParamMax=[]  DParamMin=[]  DParamMax=[]  NParamMin=[]  NParamMax=[]  KbParamMin=[]  KbParamMax=[]  KtParamMin=[]  KtParamMax=[]  KbOutMin=[]  KbOutMax=[]  KtOutMin=[]  KtOutMax=[]  IntegratorOutMin=[]  IntegratorOutMax=[]  FilterOutMin=[]  FilterOutMax=[]  SumI1OutMin=[]  SumI1OutMax=[]  SumI2OutMin=[]  SumI2OutMax=[]  SumI3OutMin=[]  SumI3OutMax=[]  SumI4OutMin=[]  SumI4OutMax=[]  SumDOutMin=[]  SumDOutMax=[]  DifferentiatorOutMin=[]  DifferentiatorOutMax=[]  FilterDiffOutCoefMin=[]  FilterDiffOutCoefMax=[]  ReciprocalOutMin=[]  ReciprocalOutMax=[]  SumDenOutMin=[]  SumDenOutMax=[]  SumNumOutMin=[]  SumNumOutMax=[]  DivideOutMin=[]  DivideOutMax=[]  UdiffTsProdOutMin=[]  UdiffTsProdOutMax=[]  NTsProdOutMin=[]  NTsProdOutMax=[]  UintegralTsProdOutMin=[]  UintegralTsProdOutMax=[]  UngainTsProdOutMin=[]  UngainTsProdOutMax=[]  IntegratorContinuousStateAttributes=''  IntegratorStateMustResolveToSignalObject=off  IntegratorRTWStateStorageClass=Auto  FilterContinuousStateAttributes=''  FilterStateMustResolveToSignalObject=off  FilterRTWStateStorageClass=Auto  ParallelPVariant=ExternalParameters  IdealPVariant=Disabled  IVariant=ExternalParameters  DVariant=ExternalParameters  IntegratorVariant=Discrete  SatVariant=Disabled  AWVariant=Passthrough  PCopyVariant=Disabled  TRVariant=Disabled  FdbkBlocksVariant=Forward  IdealPFdbkVariant=Disabled  SatFdbkVariant=Disabled  DerivativeFilterVariant=ForwardEulerFilter  NVariant=ExternalParameters  NCopyVariant=Disabled  FilterICVariant=InternalICsFilter  IntegratorICVariant=InternalICs  ExternalResetVariant=ExternalReset  TRSumVariant=Passthrough  SumFdbkVariant=Disabled  SumVariant=Sum_PID  TsampFilterVariant=InternalTs  TsampNgainVariant=Passthrough  TsampIntegralVariant=Passthrough  ExternalSaturationOutDataTypeStr=Inherit: Same as second input  aMode=0
  Relational Operator : RelationalOperator  Operator=<=  OutDataTypeStr=boolean  RndMeth=Simplest  InputSameDT=off
  Relational Operator1 : RelationalOperator  OutDataTypeStr=boolean  RndMeth=Simplest  InputSameDT=off
  Relational Operator2 : RelationalOperator  Operator===  OutDataTypeStr=boolean  RndMeth=Simplest  InputSameDT=off
  Relational Operator3 : RelationalOperator  OutDataTypeStr=boolean  RndMeth=Simplest  InputSameDT=off
  Saturation : Saturate  UpperLimit=1  LowerLimit=-1
  Scope : Scope  NumInputPorts=2
  Switch2 : Switch  Criteria=u2 ~= 0  SaturateOnIntegerOverflow=off  InputSameDT=off
  Switch3 : Switch  Criteria=u2 ~= 0  SaturateOnIntegerOverflow=off  InputSameDT=off
  Switch4 : Switch  SaturateOnIntegerOverflow=off  InputSameDT=off
  Switch5 : Switch  Criteria=u2 ~= 0  SaturateOnIntegerOverflow=off  InputSameDT=off
  Switch6 : Switch  Threshold=-2.5  SaturateOnIntegerOverflow=off  InputSameDT=off
  throttle : Outport
  wires:
  Constant2/1 -> Switch2/3
  ACC_STATUSt1/1 -> Add2/1, [accs]
  [accs] -> Add3/1
  Switch5/1 -> Switch6/1
  Constant9/1 -> Add2/2
  Switch4/1 -> Switch5/3
  In1/1 -> Gain9/1, [delta_v], Saturation/1, Abs/1
  [delta_v] -> Gain11/1
  Constant/1 -> PID Controller1/5
  Constant10/1 -> Switch6/3
  Relational Operator/1 -> Switch3/2
  Gain9/1 -> 1-D Lookup Table1/1, Switch4/2
  Constant16/1 -> Switch4/3
  1-D Lookup Table1/1 -> Switch4/1
  Abs/1 -> Gain/1
  Switch2/1 -> Switch3/1
  Switch3/1 -> PID Controller1/3
  Add3/1 -> Switch5/2
  Constant13/1 -> Switch2/1
  Gain/1 -> Relational Operator/1
  Switch6/1 -> Display/1, PID Controller1/2
  Constant17/1 -> Switch3/3
  Constant12/1 -> Switch5/1
  Constant15/1 -> Relational Operator/2
  Constant11/1 -> Add3/2
  Saturation/1 -> Scope/1, PID Controller1/1
  Gain11/1 -> Switch6/2
  Constant7/1 -> PID Controller1/4
  PID Controller1/1 -> Scope/2, Display1/1, throttle/1  "throttle"
  Add2/1 -> [status]
  [status] -> Switch2/2
  AND/1 -> PID Controller1/6
  Constant3/1 -> Relational Operator2/2
  [status] -> Relational Operator2/1
  Relational Operator2/1 -> AND/2
  Constant4/1 -> Relational Operator3/2
  [delta_v] -> Relational Operator3/1
  dec_m/1 -> Relational Operator1/1
  Constant1/1 -> Relational Operator1/2
  Relational Operator1/1 -> AND/1

== system ALL_JP360_DBW_V6_5_1103/ACC_Control/ACC_FUNCTION/Subsystem2/Limit/acceleration_throttle——PID/Out_PID ==
  note: 仪表盘速度，3pid分段
  note: 设定车速，状态机，12分段
  note: 设定车速，ifelse，12分段（可选IC速度）
  acce : Inport
  IC_V_kph : Inport  Port=2
  setvalue : Inport  Port=3
  101-110 : Subsystem
  111-120 : Subsystem
  121-130 : Subsystem
  30-1 : Subsystem
  30-40 : Subsystem
  30-50 : Subsystem
  41-50 : Subsystem
  51-60 : Subsystem
  51-80 : Subsystem
  61-70 : Subsystem
  71-80 : Subsystem
  81-90 : Subsystem
  91-100 : Subsystem
  Constant : Constant  OutDataTypeStr=int8
  Data Type Conversion : DataTypeConversion  OutDataTypeStr=double  SaturateOnIntegerOverflow=off  RndMeth=Floor
  Data Type Conversion1 : DataTypeConversion  OutDataTypeStr=single  SaturateOnIntegerOverflow=off  RndMeth=Floor
  Data Type Conversion2 : DataTypeConversion  OutDataTypeStr=single  SaturateOnIntegerOverflow=off  RndMeth=Floor
  Demux1 : Demux  Outputs=2
  Demux2 : Demux  Outputs=2
  Display : Display
  Display1 : Display
  Display2 : Display
  Gain : Gain  Gain=1/3.6
  If1 : If  NumInputs=2  IfExpression=u1>=81&u2>10  ElseIfExpressions=u1>=51&u1<=80&u2>10,u1<=50&u2>10,u2==0  ShowElse=off
  If2 : If  IfExpression=u1>0
  If3 : If  IfExpression=u1>39&u1<42  ElseIfExpressions=u1>36.3&u1<39,u1>33.5&u1<36.2,u1>30.7&u1<33.4,u1>28&u1<30.7,u1>25.2&u1<27.9,u1>22.3&u1<25.1,u1>19.5&u1<22.3,u1>16.9&u1<=19.5,u1>14&u1<16.8,u1>11.2&u1<13.9,u1>8.3&u1<11.2
  Manual Switch : ManualSwitch
  Merge1 : Merge  Inputs=4
  Merge2 : Merge
  Merge3 : Merge  Inputs=13
  Mux{,1..5} (6 alike) : Mux  Inputs=2
  Radio Button : RadioButtonGroup  LabelPosition=Hide  SelectedLabel=3pid  ButtonGroupName=Group
      settings: Values={{'3pid', '1pid(stateflow)', '12pid'}, [1 2 3]}
  Saturation : Saturate  Commented=through  UpperLimit=1000  LowerLimit=30
  Subsystem : Subsystem
  Subsystem1 : Subsystem
  Subsystem11 : Subsystem
  Subsystem12 : Subsystem
  Subsystem13 : Subsystem
  Subsystem2 : Subsystem
  up81 : Subsystem
  throttle[a]1 : Outport
  wires:
  Demux2/2 -> Display2/1
  Merge2/1 -> Demux2/1
  Demux1/2 -> Display1/1
  Merge1/1 -> Demux1/1
  Manual Switch/1 -> Gain/1
  Data Type Conversion2/1 -> Manual Switch/2
  Data Type Conversion1/1 -> Manual Switch/1
  [IC_V] -> Data Type Conversion2/1
  Subsystem/1(data) -> Saturation/1
  Constant/1 -> Subsystem/1(In1)
  Gain/1 -> If3/1
  Merge3/1 -> Subsystem/4(In4)
  [setV] -> Data Type Conversion1/1
  If3/7 -> 81-90/Action
  If3/5 -> 101-110/Action
  If3/13 -> Subsystem13/Action
  91-100/1(Out1) -> Merge3/6
  41-50/1(Out1) -> Merge3/11
  If3/4 -> 111-120/Action
  If3/12 -> 30-40/Action
  [acccc] -> 41-50/1(acce)
  30-40/1(Out1) -> Merge3/12
  [acccc] -> 71-80/1(acce)
  If3/2 -> Subsystem12/Action
  If3/9 -> 61-70/Action
  [acccc] -> 121-130/1(acce)
  [acccc] -> 91-100/1(acce)
  If3/6 -> 91-100/Action
  111-120/1(Out1) -> Merge3/4
  If3/3 -> 121-130/Action
  If3/10 -> 51-60/Action
  [acccc] -> Subsystem11/1(acce)
  Subsystem12/1(Out1) -> Merge3/2
  121-130/1(Out1) -> Merge3/3
  [acccc] -> 61-70/1(acce)
  51-60/1(Out1) -> Merge3/10
  Subsystem13/1(Out1) -> Merge3/13
  [acccc] -> 51-60/1(acce)
  If3/11 -> 41-50/Action
  [acccc] -> 101-110/1(acce)
  If3/8 -> 71-80/Action
  [acccc] -> 111-120/1(acce)
  [acccc] -> Subsystem12/1(acce)
  [acccc] -> 30-40/1(acce)
  61-70/1(Out1) -> Merge3/9
  71-80/1(Out1) -> Merge3/8
  81-90/1(Out1) -> Merge3/7
  101-110/1(Out1) -> Merge3/5
  [acccc] -> 81-90/1(acce)
  If3/1 -> Subsystem11/Action
  Subsystem11/1(Out1) -> Merge3/1
  Demux1/1 -> Subsystem/2(throttle)  "throttle"
  Demux2/1 -> Subsystem/3(In3)  "throttle"
  Mux4/1 -> Merge2/2
  Mux5/1 -> Merge2/1
  [setV] -> If2/1
  [IC_V] -> 30-1/2(IVC)
  30-1/2(Out2) -> Mux5/2
  30-1/1(Out1) -> Mux5/1
  If2/1 -> 30-1/Action
  [acccc] -> 30-1/1(acc)
  If2/2 -> Subsystem2/Action
  Subsystem2/1(Out1) -> Mux4/1
  Subsystem2/2(Out2) -> Mux4/2
  Mux3/1 -> Merge1/4
  Mux2/1 -> Merge1/3
  Mux/1 -> Merge1/1
  Mux1/1 -> Merge1/2
  Subsystem1/2(Out2) -> Mux3/2
  Subsystem1/1(Out1) -> Mux3/1
  30-50/1(Out1) -> Mux2/1
  30-50/2(Out2) -> Mux2/2
  51-80/2(Out2) -> Mux1/2
  51-80/1(Out1) -> Mux1/1
  up81/2(Out2) -> Mux/2
  up81/1(Out1) -> Mux/1
  If1/4 -> Subsystem1/Action
  setvalue/1 -> If1/2, [setV]
  Saturation/1 -> throttle[a]1/1, Display/1  "throttle"
  IC_V_kph/1 -> If1/1, [IC_V]
  acce/1 -> Data Type Conversion/1  "err_v"
  If1/3 -> 30-50/Action
  [acccc] -> 30-50/1(acce)
  If1/2 -> 51-80/Action
  If1/1 -> up81/Action
  Data Type Conversion/1 -> [acccc]
  [acccc] -> up81/1(acce)
  [acccc] -> 51-80/1(acce)

== system ALL_JP360_DBW_V6_5_1103/ACC_Control/ACC_FUNCTION/Subsystem2/Limit/acceleration_throttle——PID/Subsystem1 ==
  Action Port : ActionPort  InitializeStates=reset  PropagateVarSize=During execution
  Constant3 : Constant  Value=25  OutDataTypeStr=uint8
  Data Type Conversion : DataTypeConversion  OutDataTypeStr=single  SaturateOnIntegerOverflow=off  RndMeth=Floor
  Out1 : Outport
  wires:
  Constant3/1 -> Data Type Conversion/1  "throttle"
  Data Type Conversion/1 -> Out1/1

== system ALL_JP360_DBW_V6_5_1103/ACC_Control/ACC_FUNCTION/Subsystem2/Limit/acceleration_throttle——PID/Subsystem2 ==
  acce : Inport
  setv : Inport  Port=2
  Action Port : ActionPort  InitializeStates=reset  PropagateVarSize=During execution
  30-50 : Subsystem
  51-80 : Subsystem
  Data Type Conversion : DataTypeConversion  OutDataTypeStr=double  SaturateOnIntegerOverflow=off  RndMeth=Floor
  Data Type Conversion1 : DataTypeConversion  OutDataTypeStr=single  SaturateOnIntegerOverflow=off  RndMeth=Floor
  Demux : Demux  Outputs=2
  Display : Display
  If1 : If  IfExpression=u1>=81  ElseIfExpressions=u1>=51&u1<=80,u1<=50  ShowElse=off
  Merge1 : Merge  Inputs=3
  Mux : Mux  Inputs=2
  Mux1 : Mux  Inputs=2
  Mux2 : Mux  Inputs=2
  up81 : Subsystem
  Out1 : Outport
  wires:
  Data Type Conversion1/1 -> Out1/1
  Demux/2 -> Display/1
  Demux/1 -> Data Type Conversion1/1
  Merge1/1 -> Demux/1  "throttle"
  30-50/2(Out2) -> Mux2/2
  30-50/1(Out1) -> Mux2/1
  Mux2/1 -> Merge1/3
  51-80/1(Out1) -> Mux1/1
  Mux1/1 -> Merge1/2
  Mux/1 -> Merge1/1
  up81/1(Out1) -> Mux/1
  up81/2(Out2) -> Mux/2
  51-80/2(Out2) -> Mux1/2
  Data Type Conversion/1 -> [acccc]
  If1/1 -> up81/Action
  If1/2 -> 51-80/Action
  If1/3 -> 30-50/Action
  [acccc] -> up81/1(acce)
  [acccc] -> 30-50/1(acce)
  [acccc] -> 51-80/1(acce)
  acce/1 -> Data Type Conversion/1  "err_v"
  setv/1 -> If1/1

== system ALL_JP360_DBW_V6_5_1103/ACC_Control/ACC_FUNCTION/Subsystem2/ACC_model/TIS1 ACC action/Subsystem1/collision ==
  Action Port : ActionPort  InitializeStates=reset  PropagateVarSize=During execution  ActionPortLabel=if(u1 > 0)
  constant : Constant  Value=0  OutDataTypeStr=single
  constant1 : Constant  Value=-6  OutDataTypeStr=single
  constant2 : Constant  OutDataTypeStr=single
  acceleration [a] : Outport  InitialOutput=[0]
  deceleration [-a] : Outport  Port=2  InitialOutput=[150]
  ACC_MODE : Outport  Port=3  InitialOutput=[150]
  wires:
  constant1/1 -> deceleration [-a]/1
  constant/1 -> acceleration [a]/1
  constant2/1 -> ACC_MODE/1

== system ALL_JP360_DBW_V6_5_1103/ACC_Control/ACC_FUNCTION/Subsystem2/ACC_model/TIS1 ACC action/Subsystem1/mode change ==
  cc_throttle : Inport
  cc_brake : Inport  Port=2
  acc_obj_detected : Inport  Port=3
  a_zero : Inport  Port=4
  v_obj : Inport  Port=5
  v_set : Inport  Port=6  LockScale=on
  v_ego : Inport  Port=7
  delta_d_ego : Inport  Port=8
  dx : Inport  Port=9
  Action Port : ActionPort  InitializeStates=reset  PropagateVarSize=During execution  ActionPortLabel=else
  Chart1 : Stateflow chart  TreatAsAtomicUnit=on
      settings: PortSchema="{\"entries\":[{\"content\":{\"sides\":[{\"content\":{\"connectorIds\":[\"In1\",\"In3\",\"In2\"]},\"type\":\"ConnectorPlacement.EquallySpacedRectSide\",\"uuid\":\"a1ea63d3-d60a-460d-bbc1-1bfef8c0288a\"},{\"content\":{\"connectorIds\":[\"Out1\"],\"side\":\"RIGHT\"},\"type\":\"ConnectorPlacement.EquallySpacedRectSide\",\"uuid\":\"c1973d49-ef12-4d82-bde3-89be47febb9b\"},{\"content\":{\"connectorIds\":[],\"side\":\"TOP\"},\"type\":\"ConnectorPlacement.EquallySpacedRectSide\",\"uuid\":\"7d8c7564-58f8-4cff-9ab8-be78f521a8c3\"}]},\"type\":\"ConnectorPlacement.EquallySpacedConnector\",\"uuid\":\"5e34bcad-cbf5-413a-b462-ddd7cae783c7\"}],\"packageUris\":[\"http://schema.mathworks.com/mf0/Connector/R2020b\"],\"version\":\"1.0\"}"
  Demux : Demux  Outputs=3
  Merge : Merge
  Mux : Mux  Inputs=3
  Mux2 : Mux  Inputs=3
  cc : Subsystem  TreatAsAtomicUnit=on
  cc and close and follow : Subsystem  TreatAsAtomicUnit=on
  if : If
  acceleration [a] : Outport
  deceleration [-a] : Outport  Port=2
  ACC_MODE : Outport  Port=3
  standstill_req : Outport  Port=4  InitialOutput=[150]
  wires:
  Demux/2 -> deceleration [-a]/1
  Mux/1 -> Merge/1
  if/2 -> cc and close and follow/Action
  Demux/1 -> acceleration [a]/1
  cc/2(deceleration [-a]) -> Mux/2
  if/1 -> cc/Action
  Merge/1 -> Demux/1
  Mux2/1 -> Merge/2
  cc and close and follow/1(acceleration [a]) -> Mux2/1
  cc/1(acceleration [a]) -> Mux/1
  cc and close and follow/2(deceleration [-a]) -> Mux2/2
  Chart1/1(y) -> if/1
  acc_obj_detected/1 -> Chart1/1(acc_obj_detected)
  a_zero/1 -> cc and close and follow/1(a_zero)
  v_ego/1 -> cc and close and follow/3(v_ego)
  cc_throttle/1 -> cc and close and follow/4(cc_throttle), cc/1(throttle_in)
  cc_brake/1 -> cc and close and follow/5(cc_brake), cc/2(brake_in)
  v_obj/1 -> Chart1/2(v_obj), cc and close and follow/2(v_obj)
  delta_d_ego/1 -> cc and close and follow/6(delta_d_ego)
  cc/3(ACC_MODE) -> Mux/3
  cc and close and follow/3(ACC_MODE) -> Mux2/3
  Demux/3 -> ACC_MODE/1
  cc and close and follow/4(standstill_req) -> standstill_req/1
  v_set/1 -> Chart1/3(v_set)
  dx/1 -> cc and close and follow/7(dx)
